simulink model "CoME_ShutOff"  (R2016b)
settings: configuration reference "CodeGenConfigSet" (kept outside this file)
values from neighbouring files (symbols this model uses):
  CoME_drPedHi_C = Calibration.Parameter    [init_CoME_ShutOff.m]    (also in init_CoME_ShutOff_SIL.m = Simulink.Parameter)
  CoME_drPedLo_C = Calibration.Parameter    [init_CoME_ShutOff.m]    (also in init_CoME_ShutOff_SIL.m = Simulink.Parameter)
  CoME_nEng1Hi_C = Calibration.Parameter    [init_CoME_ShutOff.m]    (also in init_CoME_ShutOff_SIL.m = Simulink.Parameter)
  CoME_nEng1Lo_C = Calibration.Parameter    [init_CoME_ShutOff.m]    (also in init_CoME_ShutOff_SIL.m = Simulink.Parameter)
  CoME_nEng2Hi_C = Calibration.Parameter    [init_CoME_ShutOff.m]    (also in init_CoME_ShutOff_SIL.m = Simulink.Parameter)
  CoME_nEng2Lo_C = Calibration.Parameter    [init_CoME_ShutOff.m]    (also in init_CoME_ShutOff_SIL.m = Simulink.Parameter)
  CoME_numTraGearMax_C = Calibration.Parameter    [init_CoME_ShutOff.m]    (also in init_CoME_ShutOff_SIL.m = Simulink.Parameter)
  CoME_pEnv1Hi_C = Calibration.Parameter    [init_CoME_ShutOff.m]    (also in init_CoME_ShutOff_SIL.m = Simulink.Parameter)
  CoME_pEnv1Lo_C = Calibration.Parameter    [init_CoME_ShutOff.m]    (also in init_CoME_ShutOff_SIL.m = Simulink.Parameter)
  CoME_pEnv2Hi_C = Calibration.Parameter    [init_CoME_ShutOff.m]    (also in init_CoME_ShutOff_SIL.m = Simulink.Parameter)
  CoME_pEnv2Lo_C = Calibration.Parameter    [init_CoME_ShutOff.m]    (also in init_CoME_ShutOff_SIL.m = Simulink.Parameter)
  CoME_rPedHi_C = Calibration.Parameter    [init_CoME_ShutOff.m]    (also in init_CoME_ShutOff_SIL.m = Simulink.Parameter)
  CoME_rPedLo_C = Calibration.Parameter    [init_CoME_ShutOff.m]    (also in init_CoME_ShutOff_SIL.m = Simulink.Parameter)
  CoME_stAlt_CW = Calibration.Parameter    [init_CoME_ShutOff.m]    (also in init_CoME_ShutOff_SIL.m = Simulink.Parameter)
  CoME_stEEM_C = Calibration.Parameter    [init_CoME_ShutOff.m]    (also in init_CoME_ShutOff_SIL.m = Simulink.Parameter)
  CoME_stFan_CW = Calibration.Parameter    [init_CoME_ShutOff.m]    (also in init_CoME_ShutOff_SIL.m = Simulink.Parameter)
  CoME_tEnvAir1Hi_C = Calibration.Parameter    [init_CoME_ShutOff.m]    (also in init_CoME_ShutOff_SIL.m = Simulink.Parameter)
  CoME_tEnvAir1Lo_C = Calibration.Parameter    [init_CoME_ShutOff.m]    (also in init_CoME_ShutOff_SIL.m = Simulink.Parameter)
  CoME_tEnvAir2Hi_C = Calibration.Parameter    [init_CoME_ShutOff.m]    (also in init_CoME_ShutOff_SIL.m = Simulink.Parameter)
  CoME_tEnvAir2Lo_C = Calibration.Parameter    [init_CoME_ShutOff.m]    (also in init_CoME_ShutOff_SIL.m = Simulink.Parameter)
  CoME_tiBattVltgOff_C = Calibration.Parameter    [init_CoME_ShutOff.m]    (also in init_CoME_ShutOff_SIL.m = Simulink.Parameter)
  CoME_tiDrvOn_C = Calibration.Parameter    [init_CoME_ShutOff.m]    (also in init_CoME_ShutOff_SIL.m = Simulink.Parameter)
  CoME_tiMaxOffAcc_CUR = Calibration.Parameter    [init_CoME_ShutOff.m]    (also in init_CoME_ShutOff_SIL.m = Simulink.Parameter)
  CoME_tiMaxOffAcc_CURX = Calibration.Parameter    [init_CoME_ShutOff.m]    (also in init_CoME_ShutOff_SIL.m = Simulink.Parameter)
  CoME_tiMaxOffDrvOff_CUR = Calibration.Parameter    [init_CoME_ShutOff.m]    (also in init_CoME_ShutOff_SIL.m = Simulink.Parameter)
  CoME_tiMaxOffDrvOff_CURX = Calibration.Parameter    [init_CoME_ShutOff.m]    (also in init_CoME_ShutOff_SIL.m = Simulink.Parameter)
  CoME_tiMinOffAcc_CUR = Calibration.Parameter    [init_CoME_ShutOff.m]    (also in init_CoME_ShutOff_SIL.m = Simulink.Parameter)
  CoME_tiMinOffAcc_CURX = Calibration.Parameter    [init_CoME_ShutOff.m]    (also in init_CoME_ShutOff_SIL.m = Simulink.Parameter)
  CoME_tiMinOffDrvOff_CUR = Calibration.Parameter    [init_CoME_ShutOff.m]    (also in init_CoME_ShutOff_SIL.m = Simulink.Parameter)
  CoME_tiMinOffDrvOff_CURX = Calibration.Parameter    [init_CoME_ShutOff.m]    (also in init_CoME_ShutOff_SIL.m = Simulink.Parameter)
  CoME_tiOffStrtAC_C = Calibration.Parameter    [init_CoME_ShutOff.m]    (also in init_CoME_ShutOff_SIL.m = Simulink.Parameter)
  CoME_tiOffStrtAlt_C = Calibration.Parameter    [init_CoME_ShutOff.m]    (also in init_CoME_ShutOff_SIL.m = Simulink.Parameter)
  CoME_trqAcc_C = Calibration.Parameter    [init_CoME_ShutOff.m]    (also in init_CoME_ShutOff_SIL.m = Simulink.Parameter)
  CoME_trqACMax_C = Calibration.Parameter    [init_CoME_ShutOff.m]    (also in init_CoME_ShutOff_SIL.m = Simulink.Parameter)
  CoME_trqBattVltg_C = Calibration.Parameter    [init_CoME_ShutOff.m]    (also in init_CoME_ShutOff_SIL.m = Simulink.Parameter)
  CoME_trqDrvOff_C = Calibration.Parameter    [init_CoME_ShutOff.m]    (also in init_CoME_ShutOff_SIL.m = Simulink.Parameter)
  CoME_trqStrt_C = Calibration.Parameter    [init_CoME_ShutOff.m]    (also in init_CoME_ShutOff_SIL.m = Simulink.Parameter)
  CoME_uBattMinHi_C = Calibration.Parameter    [init_CoME_ShutOff.m]    (also in init_CoME_ShutOff_SIL.m = Simulink.Parameter)
  CoME_uBattMinLo_C = Calibration.Parameter    [init_CoME_ShutOff.m]    (also in init_CoME_ShutOff_SIL.m = Simulink.Parameter)
  CoME_vX1Hi_C = Calibration.Parameter    [init_CoME_ShutOff.m]    (also in init_CoME_ShutOff_SIL.m = Simulink.Parameter)
  CoME_vX1Lo_C = Calibration.Parameter    [init_CoME_ShutOff.m]    (also in init_CoME_ShutOff_SIL.m = Simulink.Parameter)
  CoME_vX2Hi_C = Calibration.Parameter    [init_CoME_ShutOff.m]    (also in init_CoME_ShutOff_SIL.m = Simulink.Parameter)
  CoME_vX2Lo_C = Calibration.Parameter    [init_CoME_ShutOff.m]    (also in init_CoME_ShutOff_SIL.m = Simulink.Parameter)
  NUM_WAHT_SY = uint8(0)    [init_CoME_ShutOff.m]    (also in init_CoME_ShutOff_SIL.m)
undefined symbols (not defined in the file or in its folder): CoME_ShutOff_DT, EngState_conv, HPUn_etaPmp_MAPY
libraries: CXLib x32, simulink x8
settings Model: Creator=Colin  LastModifiedBy=wangrui
settings ConfigSetRef: SourceLocation=Base Workspace

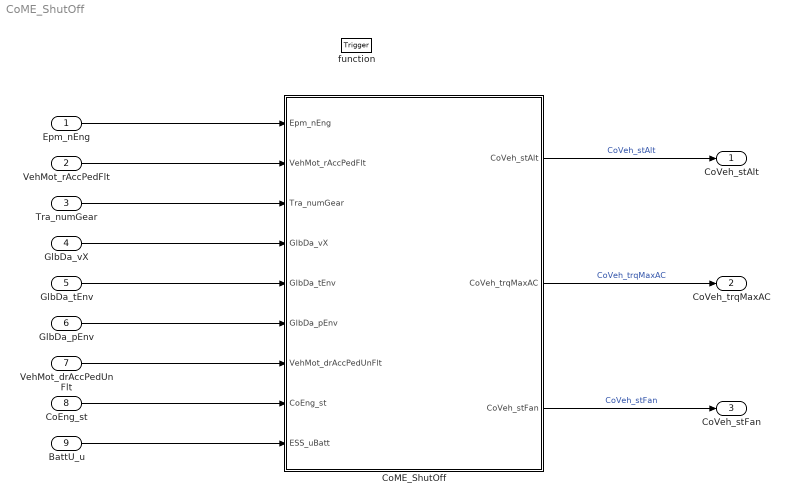
== system CoME_ShutOff ==
  Epm_nEng : Inport  Tag=rpm  Description=Engine speed  OutMin=0  OutMax=6000  OutDataTypeStr=EngSpeed_rpm
  VehMot_rAccPedFlt : Inport  Tag=%  Description=Filtered accelerator pedal value  Port=2  OutMin=0  OutMax=100  OutDataTypeStr=Accpedal_rate
  Tra_numGear : Inport  Description=Current gear information  Port=3  OutMin=-128  OutMax=127  OutDataTypeStr=Tra_num
  GlbDa_vX : Inport  Tag=km/h  Description=Longitudinal vehicle speed (X-direction)  Port=4  OutMin=0  OutMax=250  OutDataTypeStr=VehSpeed_km_h
  GlbDa_tEnv : Inport  Tag=deg  Description=environment temperature  Port=5  OutMin=-50  OutMax=150  OutDataTypeStr=Temp_deg
  GlbDa_pEnv : Inport  Tag=kPa  Description=environmental pressure  Port=6  OutMin=-3000  OutMax=3000  OutDataTypeStr=AirPressure_kPa
  VehMot_drAccPedUnFlt : Inport  Tag=%/s  Description=accelerator pedal angle slope, unfiltered  Port=7  OutMin=-400  OutMax=399  OutDataTypeStr=Accpedal_rate_s
  CoEng_st : Inport  Description=Engine coordinator state  Port=8  OutDataTypeStr=Enum: EngState_conv
  BattU_u : Inport  Tag=mv  Description=Battery voltage  Port=9  OutMin=0  OutMax=50000  OutDataTypeStr=Battery_mv
  function : TriggerPort  TriggerType=function-call  VariantControl=Variant
  CoME_ShutOff : Subsystem  RTWFcnName=CoME_ShutOff_Co  RTWFileName=CoME_ShutOff
      settings: MinAlgLoopOccurrences=on  RTWSystemCode=Nonreusable function  RTWFcnNameOpts=User specified  RTWFileNameOpts=User specified
  CoVeh_stAlt : Outport  Description=Status: Alternator start-up  OutMin=0  OutMax=1  OutDataTypeStr=boolean
  CoVeh_trqMaxAC : Outport  Tag=Nm  Description=Maximum allowed AC torque consumption  Port=2  OutMin=-3000  OutMax=3276.7  OutDataTypeStr=Trq_Nm
  CoVeh_stFan : Outport  Description=Status: Fan start-up  Port=3  OutMin=0  OutMax=1  OutDataTypeStr=boolean
  wires:
  CoME_ShutOff/1(CoVeh_stAlt) -> CoVeh_stAlt/1  "CoVeh_stAlt"
  CoME_ShutOff/2(CoVeh_trqMaxAC) -> CoVeh_trqMaxAC/1  "CoVeh_trqMaxAC"
  CoME_ShutOff/3(CoVeh_stFan) -> CoVeh_stFan/1  "CoVeh_stFan"
  Epm_nEng/1 -> CoME_ShutOff/1(Epm_nEng)
  VehMot_rAccPedFlt/1 -> CoME_ShutOff/2(VehMot_rAccPedFlt)
  Tra_numGear/1 -> CoME_ShutOff/3(Tra_numGear)
  GlbDa_vX/1 -> CoME_ShutOff/4(GlbDa_vX)
  GlbDa_tEnv/1 -> CoME_ShutOff/5(GlbDa_tEnv)
  GlbDa_pEnv/1 -> CoME_ShutOff/6(GlbDa_pEnv)
  VehMot_drAccPedUnFlt/1 -> CoME_ShutOff/7(VehMot_drAccPedUnFlt)
  CoEng_st/1 -> CoME_ShutOff/8(CoEng_st)
  BattU_u/1 -> CoME_ShutOff/9(ESS_uBatt)

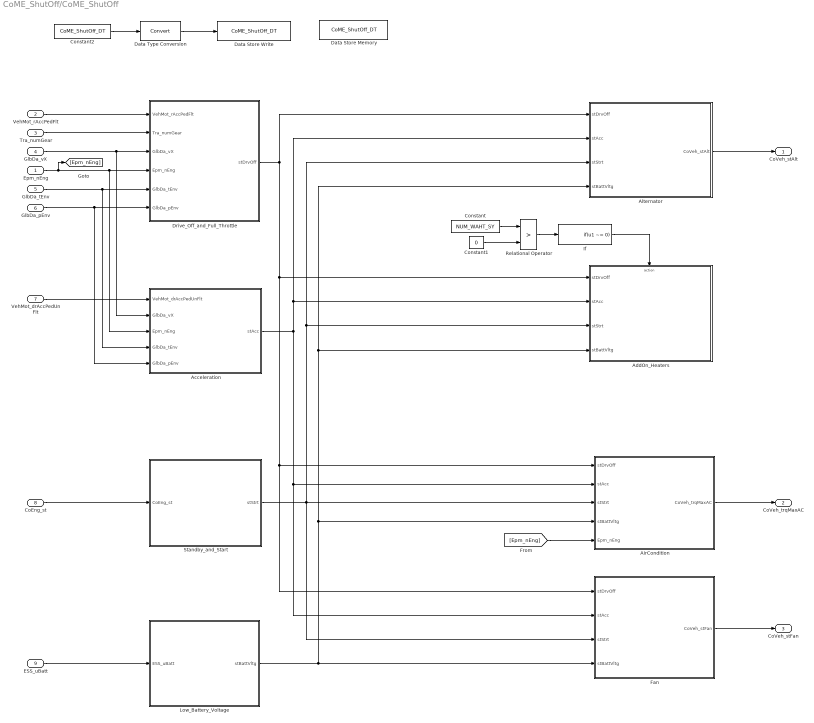
== system CoME_ShutOff/CoME_ShutOff ==
  Epm_nEng : Inport
  VehMot_rAccPedFlt : Inport  Port=2
  Tra_numGear : Inport  Port=3
  GlbDa_vX : Inport  Port=4
  GlbDa_tEnv : Inport  Port=5
  GlbDa_pEnv : Inport  Port=6
  VehMot_drAccPedUnFlt : Inport  Port=7
  CoEng_st : Inport  Port=8
  ESS_uBatt : Inport  Port=9
  Acceleration : Subsystem
  AddOn_Heaters : Subsystem  TreatAsAtomicUnit=on
  AirCondition : Subsystem
      settings: MinAlgLoopOccurrences=on
  Alternator : Subsystem
  Constant : Constant  Value=NUM_WAHT_SY  OutDataTypeStr=uint8
  Constant1 : Constant  Value=0  OutDataTypeStr=Inherit: Inherit via back propagation
  Constant2 : Constant  Value=CoME_ShutOff_DT
  Data Store Memory : DataStoreMemory  DataStoreName=CoME_ShutOff_DT  ReadBeforeWriteMsg=warning  WriteAfterWriteMsg=warning  WriteAfterReadMsg=warning  InitialValue=10  ShowAdditionalParam=off  OutDataTypeStr=EngTime_ms
  Data Store Write : DataStoreWrite  DataStoreName=CoME_ShutOff_DT
  Data Type Conversion : DataTypeConversion
  Drive_Off_and_Full_Throttle : Subsystem
  Fan : Subsystem
  If : If  IfExpression=u1 ~= 0  ShowElse=off
  Low_Battery_Voltage : Subsystem
  Relational Operator : RelationalOperator  Operator=>  OutDataTypeStr=boolean  RndMeth=Simplest  InputSameDT=on
  Standby_and_Start : Subsystem
  CoVeh_stAlt : Outport
  CoVeh_trqMaxAC : Outport  Port=2
  CoVeh_stFan : Outport  Port=3
  wires:
  Epm_nEng/1 -> [Epm_nEng], Drive_Off_and_Full_Throttle/4(Epm_nEng), Acceleration/3(Epm_nEng)
  VehMot_rAccPedFlt/1 -> Drive_Off_and_Full_Throttle/1(VehMot_rAccPedFlt)
  ESS_uBatt/1 -> Low_Battery_Voltage/1(ESS_uBatt)
  GlbDa_pEnv/1 -> Drive_Off_and_Full_Throttle/6(GlbDa_pEnv), Acceleration/5(GlbDa_pEnv)
  GlbDa_tEnv/1 -> Drive_Off_and_Full_Throttle/5(GlbDa_tEnv), Acceleration/4(GlbDa_tEnv)
  GlbDa_vX/1 -> Drive_Off_and_Full_Throttle/3(GlbDa_vX), Acceleration/2(GlbDa_vX)
  Tra_numGear/1 -> Drive_Off_and_Full_Throttle/2(Tra_numGear)
  VehMot_drAccPedUnFlt/1 -> Acceleration/1(VehMot_drAccPedUnFlt)
  AirCondition/1(CoVeh_trqMaxAC) -> CoVeh_trqMaxAC/1
  Fan/1(CoVeh_stFan) -> CoVeh_stFan/1
  CoEng_st/1 -> Standby_and_Start/1(CoEng_st)
  [Epm_nEng] -> AirCondition/5(Epm_nEng)
  Low_Battery_Voltage/1(stBattVltg) -> Fan/4(stBattVltg), AirCondition/4(stBattVltg), AddOn_Heaters/4(stBattVltg), Alternator/4(stBattVltg)
  Drive_Off_and_Full_Throttle/1(stDrvOff) -> Alternator/1(stDrvOff), AirCondition/1(stDrvOff), Fan/1(stDrvOff), AddOn_Heaters/1(stDrvOff)
  Standby_and_Start/1(stStrt) -> AirCondition/3(stStrt), AddOn_Heaters/3(stStrt), Alternator/3(stStrt), Fan/3(stStrt)
  Acceleration/1(stAcc) -> Alternator/2(stAcc), AddOn_Heaters/2(stAcc), AirCondition/2(stAcc), Fan/2(stAcc)
  Alternator/1(CoVeh_stAlt) -> CoVeh_stAlt/1
  Constant1/1 -> Relational Operator/2
  If/1 -> AddOn_Heaters/Action
  Constant/1 -> Relational Operator/1
  Relational Operator/1 -> If/1
  Constant2/1 -> Data Type Conversion/1
  Data Type Conversion/1 -> Data Store Write/1

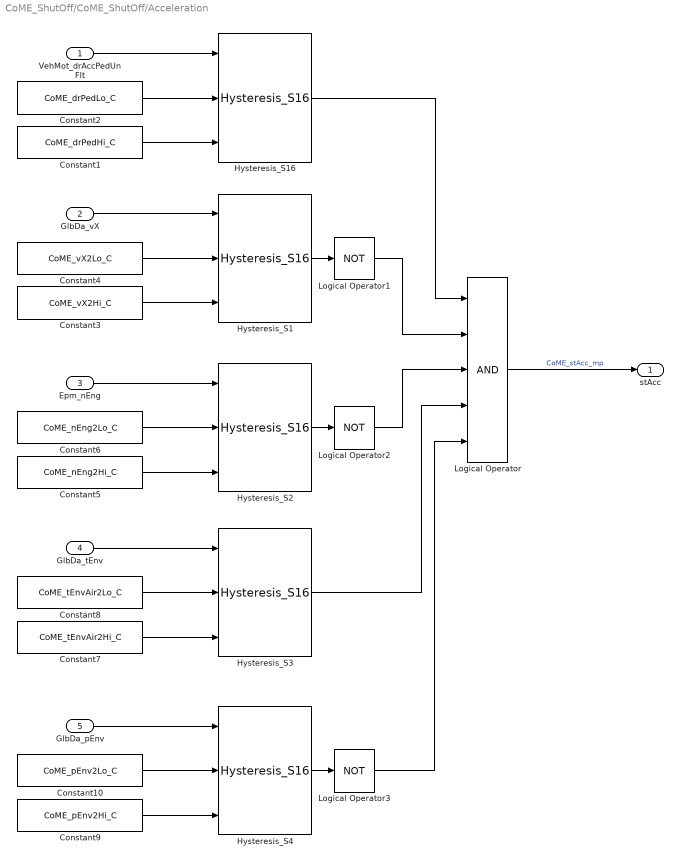
== system CoME_ShutOff/CoME_ShutOff/Acceleration ==
  VehMot_drAccPedUnFlt : Inport
  GlbDa_vX : Inport  Port=2
  Epm_nEng : Inport  Port=3
  GlbDa_tEnv : Inport  Port=4
  GlbDa_pEnv : Inport  Port=5
  Constant1 : Constant  Value=CoME_drPedHi_C
  Constant10 : Constant  Value=CoME_pEnv2Lo_C
  Constant2 : Constant  Value=CoME_drPedLo_C
  Constant3 : Constant  Value=CoME_vX2Hi_C
  Constant4 : Constant  Value=CoME_vX2Lo_C
  Constant5 : Constant  Value=CoME_nEng2Hi_C
  Constant6 : Constant  Value=CoME_nEng2Lo_C
  Constant7 : Constant  Value=CoME_tEnvAir2Hi_C
  Constant8 : Constant  Value=CoME_tEnvAir2Lo_C
  Constant9 : Constant  Value=CoME_pEnv2Hi_C
  Hysteresis_S{1..4,16} (5 alike) : CXLib/Hysteresis_S16
  Logical Operator : Logic  Inputs=5  OutDataTypeStr=boolean
  Logical Operator1 : Logic  Operator=NOT  OutDataTypeStr=boolean
  Logical Operator2 : Logic  Operator=NOT  OutDataTypeStr=boolean
  Logical Operator3 : Logic  Operator=NOT  OutDataTypeStr=boolean
  stAcc : Outport
  wires:
  Hysteresis_S16/1 -> Logical Operator/1
  Logical Operator1/1 -> Logical Operator/2
  Logical Operator2/1 -> Logical Operator/3
  Hysteresis_S3/1 -> Logical Operator/4
  Logical Operator3/1 -> Logical Operator/5
  Hysteresis_S4/1 -> Logical Operator3/1
  Hysteresis_S2/1 -> Logical Operator2/1
  Hysteresis_S1/1 -> Logical Operator1/1
  GlbDa_pEnv/1 -> Hysteresis_S4/1
  Constant10/1 -> Hysteresis_S4/2
  Constant9/1 -> Hysteresis_S4/3
  GlbDa_tEnv/1 -> Hysteresis_S3/1
  Constant8/1 -> Hysteresis_S3/2
  Constant7/1 -> Hysteresis_S3/3
  Epm_nEng/1 -> Hysteresis_S2/1
  Constant6/1 -> Hysteresis_S2/2
  Constant5/1 -> Hysteresis_S2/3
  GlbDa_vX/1 -> Hysteresis_S1/1
  Constant4/1 -> Hysteresis_S1/2
  Constant3/1 -> Hysteresis_S1/3
  Constant1/1 -> Hysteresis_S16/3
  Constant2/1 -> Hysteresis_S16/2
  VehMot_drAccPedUnFlt/1 -> Hysteresis_S16/1
  Logical Operator/1 -> stAcc/1  "CoME_stAcc_mp"

== system CoME_ShutOff/CoME_ShutOff/AddOn_Heaters ==
  note: %文档中没有图或文字描述%
  stDrvOff : Inport
  stAcc : Inport  Port=2
  stStrt : Inport  Port=3
  stBattVltg : Inport  Port=4
  Action Port : ActionPort  ActionType=then
  Terminator{,1..3} (4 alike) : Terminator
  wires:
  stBattVltg/1 -> Terminator3/1
  stStrt/1 -> Terminator2/1
  stAcc/1 -> Terminator1/1
  stDrvOff/1 -> Terminator/1

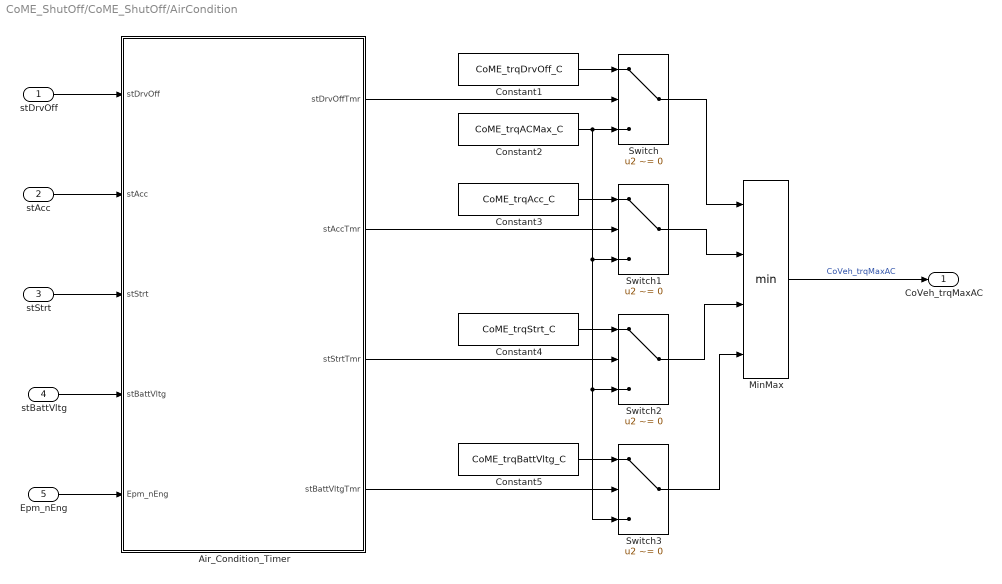
== system CoME_ShutOff/CoME_ShutOff/AirCondition ==
  stDrvOff : Inport
  stAcc : Inport  Port=2
  stStrt : Inport  Port=3
  stBattVltg : Inport  Port=4
  Epm_nEng : Inport  Port=5
  Air_Condition_Timer : Subsystem
  Constant1 : Constant  Value=CoME_trqDrvOff_C
  Constant2 : Constant  Value=CoME_trqACMax_C
  Constant3 : Constant  Value=CoME_trqAcc_C
  Constant4 : Constant  Value=CoME_trqStrt_C
  Constant5 : Constant  Value=CoME_trqBattVltg_C
  MinMax : MinMax  Inputs=4  InputSameDT=on
  Switch{,1..3} (4 alike) : Switch  Criteria=u2 ~= 0  InputSameDT=on
  CoVeh_trqMaxAC : Outport
  wires:
  Epm_nEng/1 -> Air_Condition_Timer/5(Epm_nEng)
  stDrvOff/1 -> Air_Condition_Timer/1(stDrvOff)
  stAcc/1 -> Air_Condition_Timer/2(stAcc)
  stStrt/1 -> Air_Condition_Timer/3(stStrt)
  stBattVltg/1 -> Air_Condition_Timer/4(stBattVltg)
  Air_Condition_Timer/4(stBattVltgTmr) -> Switch3/2
  Air_Condition_Timer/3(stStrtTmr) -> Switch2/2
  Air_Condition_Timer/2(stAccTmr) -> Switch1/2
  Air_Condition_Timer/1(stDrvOffTmr) -> Switch/2
  Constant5/1 -> Switch3/1
  Constant4/1 -> Switch2/1
  Constant3/1 -> Switch1/1
  Constant1/1 -> Switch/1
  Constant2/1 -> Switch/3, Switch1/3, Switch3/3, Switch2/3
  Switch/1 -> MinMax/1
  Switch1/1 -> MinMax/2
  Switch2/1 -> MinMax/3
  Switch3/1 -> MinMax/4
  MinMax/1 -> CoVeh_trqMaxAC/1  "CoVeh_trqMaxAC"

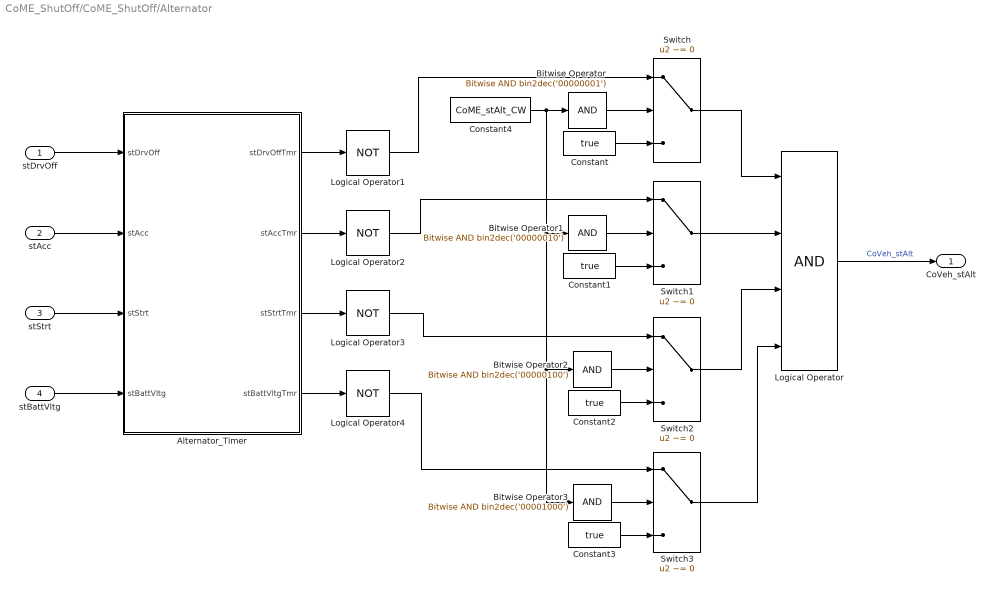
== system CoME_ShutOff/CoME_ShutOff/Alternator ==
  stDrvOff : Inport
  stAcc : Inport  Port=2
  stStrt : Inport  Port=3
  stBattVltg : Inport  Port=4
  Alternator_Timer : Subsystem
  Bitwise Operator : simulink/Logic and Bit Operations/Bitwise Operator  logicop=AND  UseBitMask=on  BitMask=bin2dec('00000001')  BitMaskRealWorld=Stored Integer
  Bitwise Operator1 : simulink/Logic and Bit Operations/Bitwise Operator  logicop=AND  UseBitMask=on  BitMask=bin2dec('00000010')  BitMaskRealWorld=Stored Integer
  Bitwise Operator2 : simulink/Logic and Bit Operations/Bitwise Operator  logicop=AND  UseBitMask=on  BitMask=bin2dec('00000100')  BitMaskRealWorld=Stored Integer
  Bitwise Operator3 : simulink/Logic and Bit Operations/Bitwise Operator  logicop=AND  UseBitMask=on  BitMask=bin2dec('00001000')  BitMaskRealWorld=Stored Integer
  Constant{,1..3} (4 alike) : Constant  Value=true  OutDataTypeStr=boolean
  Constant4 : Constant  Value=CoME_stAlt_CW
  Logical Operator : Logic  Inputs=4  OutDataTypeStr=boolean
  Logical Operator{1..4} (4 alike) : Logic  Operator=NOT  OutDataTypeStr=boolean
  Switch{,1..3} (4 alike) : Switch  Criteria=u2 ~= 0  InputSameDT=on
  CoVeh_stAlt : Outport
  wires:
  Logical Operator4/1 -> Switch3/1
  Bitwise Operator3/1 -> Switch3/2
  Logical Operator3/1 -> Switch2/1
  Bitwise Operator2/1 -> Switch2/2
  Logical Operator2/1 -> Switch1/1
  Bitwise Operator1/1 -> Switch1/2
  Logical Operator1/1 -> Switch/1
  Constant4/1 -> Bitwise Operator1/1, Bitwise Operator2/1, Bitwise Operator3/1, Bitwise Operator/1
  Bitwise Operator/1 -> Switch/2
  Constant3/1 -> Switch3/3
  Constant2/1 -> Switch2/3
  Constant1/1 -> Switch1/3
  Constant/1 -> Switch/3
  Switch3/1 -> Logical Operator/4
  Switch2/1 -> Logical Operator/3
  Switch1/1 -> Logical Operator/2
  Switch/1 -> Logical Operator/1
  Logical Operator/1 -> CoVeh_stAlt/1  "CoVeh_stAlt"
  Alternator_Timer/4(stBattVltgTmr) -> Logical Operator4/1
  Alternator_Timer/3(stStrtTmr) -> Logical Operator3/1
  Alternator_Timer/2(stAccTmr) -> Logical Operator2/1
  Alternator_Timer/1(stDrvOffTmr) -> Logical Operator1/1
  stBattVltg/1 -> Alternator_Timer/4(stBattVltg)
  stStrt/1 -> Alternator_Timer/3(stStrt)
  stAcc/1 -> Alternator_Timer/2(stAcc)
  stDrvOff/1 -> Alternator_Timer/1(stDrvOff)

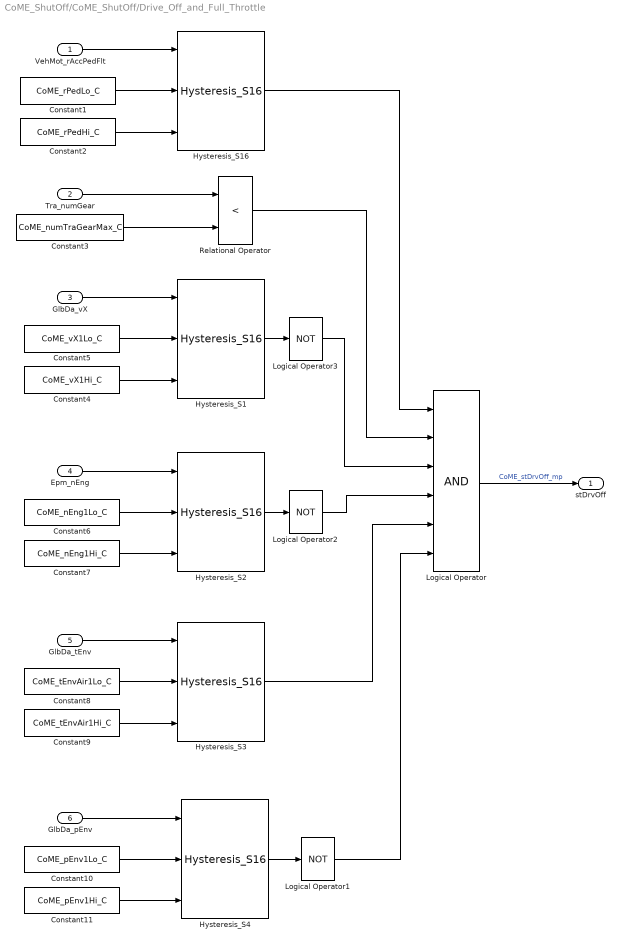
== system CoME_ShutOff/CoME_ShutOff/Drive_Off_and_Full_Throttle ==
  VehMot_rAccPedFlt : Inport
  Tra_numGear : Inport  Port=2
  GlbDa_vX : Inport  Port=3
  Epm_nEng : Inport  Port=4
  GlbDa_tEnv : Inport  Port=5
  GlbDa_pEnv : Inport  Port=6
  Constant1 : Constant  Value=CoME_rPedLo_C
  Constant10 : Constant  Value=CoME_pEnv1Lo_C
  Constant11 : Constant  Value=CoME_pEnv1Hi_C
  Constant2 : Constant  Value=CoME_rPedHi_C
  Constant3 : Constant  Value=CoME_numTraGearMax_C
  Constant4 : Constant  Value=CoME_vX1Hi_C
  Constant5 : Constant  Value=CoME_vX1Lo_C
  Constant6 : Constant  Value=CoME_nEng1Lo_C
  Constant7 : Constant  Value=CoME_nEng1Hi_C
  Constant8 : Constant  Value=CoME_tEnvAir1Lo_C
  Constant9 : Constant  Value=CoME_tEnvAir1Hi_C
  Hysteresis_S{1..4,16} (5 alike) : CXLib/Hysteresis_S16
  Logical Operator : Logic  Inputs=6  OutDataTypeStr=boolean
  Logical Operator1 : Logic  Operator=NOT  OutDataTypeStr=boolean
  Logical Operator2 : Logic  Operator=NOT  OutDataTypeStr=boolean
  Logical Operator3 : Logic  Operator=NOT  OutDataTypeStr=boolean
  Relational Operator : RelationalOperator  Operator=<  OutDataTypeStr=boolean  RndMeth=Simplest  InputSameDT=on
  stDrvOff : Outport
  wires:
  Constant10/1 -> Hysteresis_S4/2
  Constant11/1 -> Hysteresis_S4/3
  GlbDa_pEnv/1 -> Hysteresis_S4/1
  Constant9/1 -> Hysteresis_S3/3
  Constant8/1 -> Hysteresis_S3/2
  GlbDa_tEnv/1 -> Hysteresis_S3/1
  Constant7/1 -> Hysteresis_S2/3
  Constant6/1 -> Hysteresis_S2/2
  Epm_nEng/1 -> Hysteresis_S2/1
  GlbDa_vX/1 -> Hysteresis_S1/1
  Constant5/1 -> Hysteresis_S1/2
  Constant4/1 -> Hysteresis_S1/3
  Logical Operator3/1 -> Logical Operator/3
  Hysteresis_S1/1 -> Logical Operator3/1
  Logical Operator2/1 -> Logical Operator/4
  Hysteresis_S2/1 -> Logical Operator2/1
  Hysteresis_S3/1 -> Logical Operator/5
  Logical Operator1/1 -> Logical Operator/6
  Hysteresis_S4/1 -> Logical Operator1/1
  Tra_numGear/1 -> Relational Operator/1
  Constant3/1 -> Relational Operator/2
  Relational Operator/1 -> Logical Operator/2
  Constant2/1 -> Hysteresis_S16/3
  Constant1/1 -> Hysteresis_S16/2
  VehMot_rAccPedFlt/1 -> Hysteresis_S16/1
  Hysteresis_S16/1 -> Logical Operator/1
  Logical Operator/1 -> stDrvOff/1  "CoME_stDrvOff_mp"

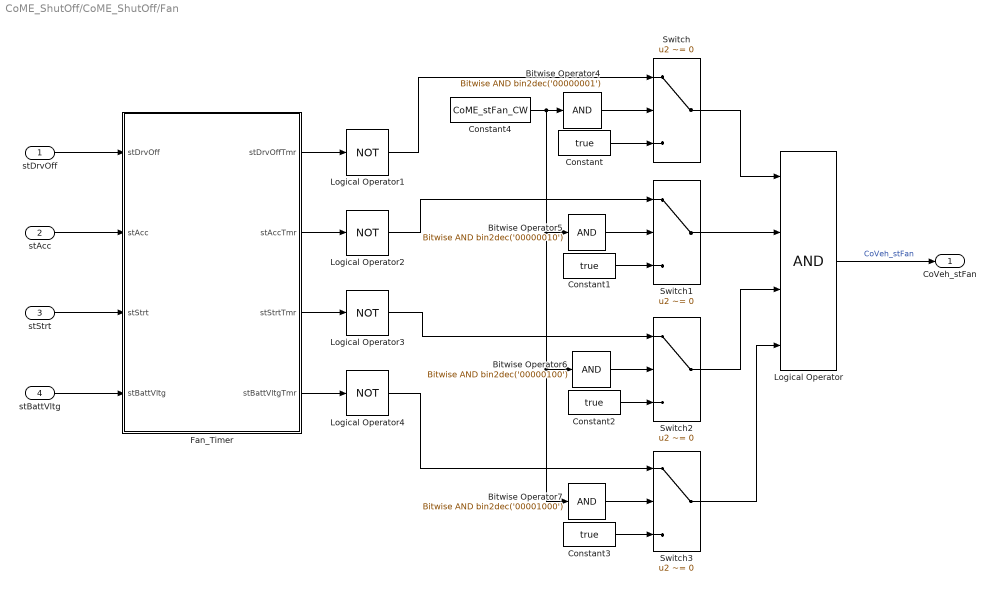
== system CoME_ShutOff/CoME_ShutOff/Fan ==
  stDrvOff : Inport
  stAcc : Inport  Port=2
  stStrt : Inport  Port=3
  stBattVltg : Inport  Port=4
  Bitwise Operator4 : simulink/Logic and Bit Operations/Bitwise Operator  logicop=AND  UseBitMask=on  BitMask=bin2dec('00000001')  BitMaskRealWorld=Stored Integer
  Bitwise Operator5 : simulink/Logic and Bit Operations/Bitwise Operator  logicop=AND  UseBitMask=on  BitMask=bin2dec('00000010')  BitMaskRealWorld=Stored Integer
  Bitwise Operator6 : simulink/Logic and Bit Operations/Bitwise Operator  logicop=AND  UseBitMask=on  BitMask=bin2dec('00000100')  BitMaskRealWorld=Stored Integer
  Bitwise Operator7 : simulink/Logic and Bit Operations/Bitwise Operator  logicop=AND  UseBitMask=on  BitMask=bin2dec('00001000')  BitMaskRealWorld=Stored Integer
  Constant{,1..3} (4 alike) : Constant  Value=true  OutDataTypeStr=boolean
  Constant4 : Constant  Value=CoME_stFan_CW
  Fan_Timer : Subsystem
  Logical Operator : Logic  Inputs=4  OutDataTypeStr=boolean
  Logical Operator{1..4} (4 alike) : Logic  Operator=NOT  OutDataTypeStr=boolean
  Switch{,1..3} (4 alike) : Switch  Criteria=u2 ~= 0  InputSameDT=on
  CoVeh_stFan : Outport
  wires:
  Logical Operator4/1 -> Switch3/1
  Bitwise Operator7/1 -> Switch3/2
  Logical Operator3/1 -> Switch2/1
  Bitwise Operator6/1 -> Switch2/2
  Logical Operator2/1 -> Switch1/1
  Bitwise Operator5/1 -> Switch1/2
  Logical Operator1/1 -> Switch/1
  Constant4/1 -> Bitwise Operator5/1, Bitwise Operator6/1, Bitwise Operator7/1, Bitwise Operator4/1
  Bitwise Operator4/1 -> Switch/2
  Constant3/1 -> Switch3/3
  Constant2/1 -> Switch2/3
  Constant1/1 -> Switch1/3
  Constant/1 -> Switch/3
  Switch3/1 -> Logical Operator/4
  Switch2/1 -> Logical Operator/3
  Switch1/1 -> Logical Operator/2
  Switch/1 -> Logical Operator/1
  Logical Operator/1 -> CoVeh_stFan/1  "CoVeh_stFan"
  Fan_Timer/4(stBattVltgTmr) -> Logical Operator4/1
  Fan_Timer/3(stStrtTmr) -> Logical Operator3/1
  Fan_Timer/2(stAccTmr) -> Logical Operator2/1
  Fan_Timer/1(stDrvOffTmr) -> Logical Operator1/1
  stBattVltg/1 -> Fan_Timer/4(stBattVltg)
  stStrt/1 -> Fan_Timer/3(stStrt)
  stAcc/1 -> Fan_Timer/2(stAcc)
  stDrvOff/1 -> Fan_Timer/1(stDrvOff)

== system CoME_ShutOff/CoME_ShutOff/Low_Battery_Voltage ==
  ESS_uBatt : Inport
  Constant1 : Constant  Value=CoME_uBattMinHi_C
  Constant2 : Constant  Value=CoME_uBattMinLo_C
  Electrical_Energy : Subsystem
  Hysteresis_S16 : CXLib/Hysteresis_S16
  Logical Operator1 : Logic  Operator=NOT  AllPortsSameDT=off  OutDataTypeStr=boolean
  stBattVltg : Outport
  wires:
  Constant1/1 -> Hysteresis_S16/3
  Constant2/1 -> Hysteresis_S16/2
  ESS_uBatt/1 -> Hysteresis_S16/1
  Electrical_Energy/1(stBattVltg) -> stBattVltg/1  "CoME_stBattVltg_mp"
  Logical Operator1/1 -> Electrical_Energy/1(stUBatt)
  Hysteresis_S16/1 -> Logical Operator1/1

== system CoME_ShutOff/CoME_ShutOff/Standby_and_Start ==
  CoEng_st : Inport
  Constant1 : Constant  Value=EngState_conv.COENG_READY
  Constant2 : Constant  Value=EngState_conv.COENG_CRANKING
  Constant3 : Constant  Value=EngState_conv.COENG_STANDBY
  Logical Operator : Logic  Operator=OR  Inputs=3  OutDataTypeStr=boolean
  Relational Operator : RelationalOperator  Operator===  OutDataTypeStr=boolean  RndMeth=Simplest  InputSameDT=on
  Relational Operator1 : RelationalOperator  Operator===  OutDataTypeStr=boolean  RndMeth=Simplest  InputSameDT=on
  Relational Operator2 : RelationalOperator  Operator===  OutDataTypeStr=boolean  RndMeth=Simplest  InputSameDT=on
  stStrt : Outport
  wires:
  Constant3/1 -> Relational Operator2/2
  Constant1/1 -> Relational Operator1/2
  Constant2/1 -> Relational Operator/2
  CoEng_st/1 -> Relational Operator/1, Relational Operator1/1, Relational Operator2/1
  Relational Operator/1 -> Logical Operator/1
  Relational Operator2/1 -> Logical Operator/3
  Relational Operator1/1 -> Logical Operator/2
  Logical Operator/1 -> stStrt/1  "CoME_stStrt_mp"

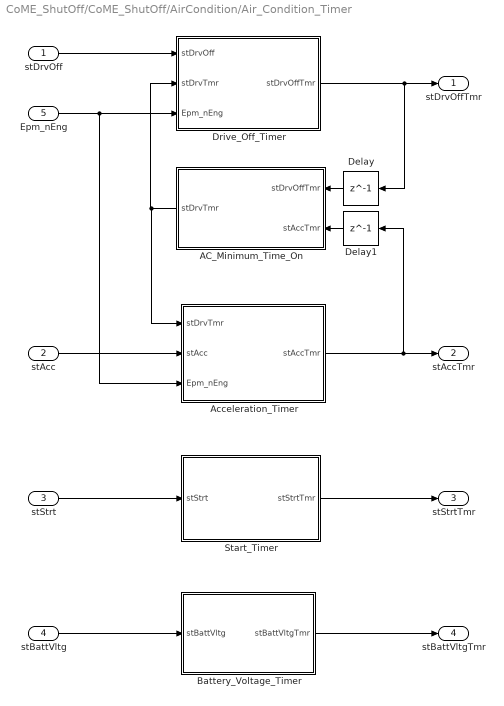
== system CoME_ShutOff/CoME_ShutOff/AirCondition/Air_Condition_Timer ==
  stDrvOff : Inport
  stAcc : Inport  Port=2
  stStrt : Inport  Port=3
  stBattVltg : Inport  Port=4
  Epm_nEng : Inport  Port=5
  AC_Minimum_Time_On : Subsystem
  Acceleration_Timer : Subsystem
  Battery_Voltage_Timer : Subsystem
  Delay : Delay  DelayLength=1  InitialCondition=0
  Delay1 : Delay  DelayLength=1  InitialCondition=0
  Drive_Off_Timer : Subsystem
  Start_Timer : Subsystem
  stDrvOffTmr : Outport
  stAccTmr : Outport  Port=2
  stStrtTmr : Outport  Port=3
  stBattVltgTmr : Outport  Port=4
  wires:
  Delay1/1 -> AC_Minimum_Time_On/2(stAccTmr)
  Delay/1 -> AC_Minimum_Time_On/1(stDrvOffTmr)
  Epm_nEng/1 -> Drive_Off_Timer/3(Epm_nEng), Acceleration_Timer/3(Epm_nEng)
  Battery_Voltage_Timer/1(stBattVltgTmr) -> stBattVltgTmr/1
  stBattVltg/1 -> Battery_Voltage_Timer/1(stBattVltg)
  stStrt/1 -> Start_Timer/1(stStrt)
  Start_Timer/1(stStrtTmr) -> stStrtTmr/1
  stAcc/1 -> Acceleration_Timer/2(stAcc)
  Acceleration_Timer/1(stAccTmr) -> Delay1/1, stAccTmr/1
  AC_Minimum_Time_On/1(stDrvTmr) -> Drive_Off_Timer/2(stDrvTmr), Acceleration_Timer/1(stDrvTmr)
  Drive_Off_Timer/1(stDrvOffTmr) -> stDrvOffTmr/1, Delay/1
  stDrvOff/1 -> Drive_Off_Timer/1(stDrvOff)

== system CoME_ShutOff/CoME_ShutOff/Alternator/Alternator_Timer ==
  stDrvOff : Inport
  stAcc : Inport  Port=2
  stStrt : Inport  Port=3
  stBattVltg : Inport  Port=4
  Constant1 : Constant  Value=1000  OutDataTypeStr=int16
  Constant2 : Constant  Value=CoME_tiOffStrtAlt_C
  Data Store Read : DataStoreRead  DataStoreName=CoME_ShutOff_DT
  Divide : Product  Inputs=**  OutDataTypeStr=EngTime_ms  SaturateOnIntegerOverflow=on
  TurnOffDelay : CXLib/TurnOffDelay
  stDrvOffTmr : Outport
  stAccTmr : Outport  Port=2
  stStrtTmr : Outport  Port=3
  stBattVltgTmr : Outport  Port=4
  wires:
  Constant1/1 -> Divide/2
  Constant2/1 -> Divide/1
  Data Store Read/1 -> TurnOffDelay/3
  stStrt/1 -> TurnOffDelay/1
  TurnOffDelay/1 -> stStrtTmr/1
  stAcc/1 -> stAccTmr/1
  stDrvOff/1 -> stDrvOffTmr/1
  stBattVltg/1 -> stBattVltgTmr/1
  Divide/1 -> TurnOffDelay/2

== system CoME_ShutOff/CoME_ShutOff/Fan/Fan_Timer ==
  stDrvOff : Inport
  stAcc : Inport  Port=2
  stStrt : Inport  Port=3
  stBattVltg : Inport  Port=4
  stDrvOffTmr : Outport
  stAccTmr : Outport  Port=2
  stStrtTmr : Outport  Port=3
  stBattVltgTmr : Outport  Port=4
  wires:
  stStrt/1 -> stStrtTmr/1
  stAcc/1 -> stAccTmr/1
  stDrvOff/1 -> stDrvOffTmr/1
  stBattVltg/1 -> stBattVltgTmr/1

== system CoME_ShutOff/CoME_ShutOff/Low_Battery_Voltage/Electrical_Energy ==
  stUBatt : Inport
  Constant2 : Constant  Value=CoME_stEEM_C
  Logical Operator : Logic  Operator=OR  OutDataTypeStr=boolean
  stBattVltg : Outport
  wires:
  Constant2/1 -> Logical Operator/2
  stUBatt/1 -> Logical Operator/1
  Logical Operator/1 -> stBattVltg/1

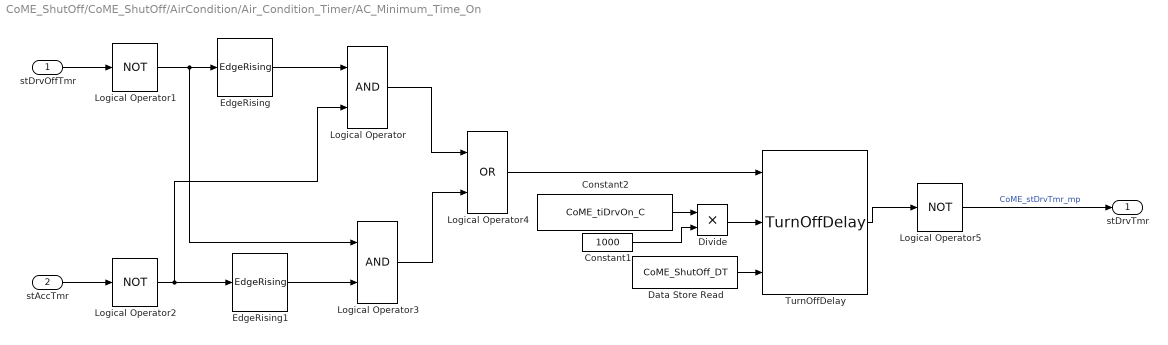
== system CoME_ShutOff/CoME_ShutOff/AirCondition/Air_Condition_Timer/AC_Minimum_Time_On ==
  stDrvOffTmr : Inport
  stAccTmr : Inport  Port=2
  Constant1 : Constant  Value=1000  OutDataTypeStr=int16
  Constant2 : Constant  Value=CoME_tiDrvOn_C
  Data Store Read : DataStoreRead  DataStoreName=CoME_ShutOff_DT
  Divide : Product  Inputs=**  OutDataTypeStr=EngTime_ms  SaturateOnIntegerOverflow=on
  EdgeRising : CXLib/EdgeRising
  EdgeRising1 : CXLib/EdgeRising
  Logical Operator : Logic  OutDataTypeStr=boolean
  Logical Operator1 : Logic  Operator=NOT  OutDataTypeStr=boolean
  Logical Operator2 : Logic  Operator=NOT  OutDataTypeStr=boolean
  Logical Operator3 : Logic  OutDataTypeStr=boolean
  Logical Operator4 : Logic  Operator=OR  OutDataTypeStr=boolean
  Logical Operator5 : Logic  Operator=NOT  OutDataTypeStr=boolean
  TurnOffDelay : CXLib/TurnOffDelay
  stDrvTmr : Outport
  wires:
  Constant1/1 -> Divide/2
  Constant2/1 -> Divide/1
  Divide/1 -> TurnOffDelay/2
  Data Store Read/1 -> TurnOffDelay/3
  Logical Operator5/1 -> stDrvTmr/1  "CoME_stDrvTmr_mp"
  TurnOffDelay/1 -> Logical Operator5/1
  Logical Operator4/1 -> TurnOffDelay/1
  Logical Operator3/1 -> Logical Operator4/2
  Logical Operator/1 -> Logical Operator4/1
  EdgeRising1/1 -> Logical Operator3/2
  Logical Operator2/1 -> Logical Operator/2, EdgeRising1/1
  stAccTmr/1 -> Logical Operator2/1
  EdgeRising/1 -> Logical Operator/1
  Logical Operator1/1 -> EdgeRising/1, Logical Operator3/1
  stDrvOffTmr/1 -> Logical Operator1/1

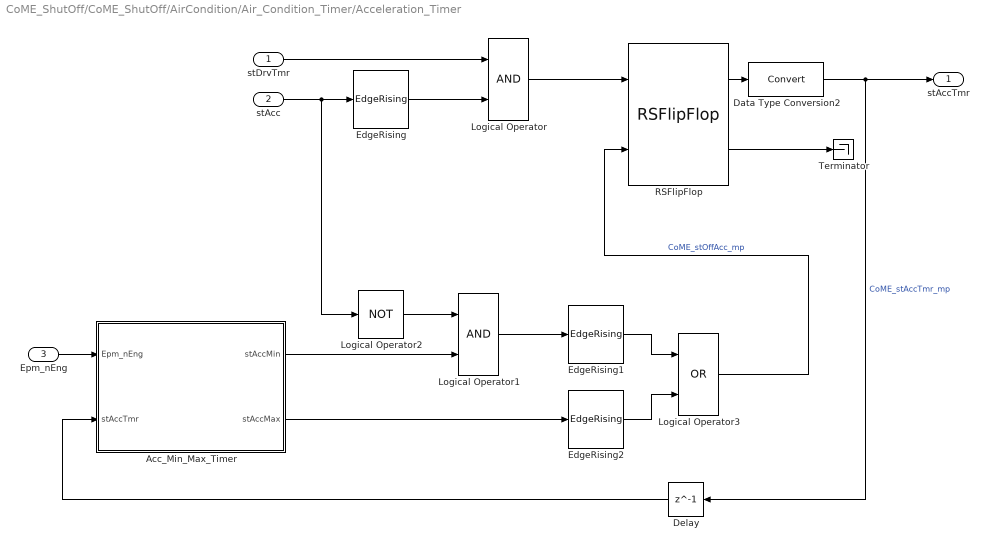
== system CoME_ShutOff/CoME_ShutOff/AirCondition/Air_Condition_Timer/Acceleration_Timer ==
  stDrvTmr : Inport
  stAcc : Inport  Port=2
  Epm_nEng : Inport  Port=3
  Acc_Min_Max_Timer : Subsystem
  Data Type Conversion2 : DataTypeConversion
  Delay : Delay  DelayLength=1  InitialCondition=0
  EdgeRising : CXLib/EdgeRising
  EdgeRising1 : CXLib/EdgeRising
  EdgeRising2 : CXLib/EdgeRising
  Logical Operator : Logic  OutDataTypeStr=boolean
  Logical Operator1 : Logic  OutDataTypeStr=boolean
  Logical Operator2 : Logic  Operator=NOT  OutDataTypeStr=boolean
  Logical Operator3 : Logic  Operator=OR  OutDataTypeStr=boolean
  RSFlipFlop : CXLib/RSFlipFlop
  Terminator : Terminator
  stAccTmr : Outport
  wires:
  Delay/1 -> Acc_Min_Max_Timer/2(stAccTmr)
  Data Type Conversion2/1 -> Delay/1, stAccTmr/1  "CoME_stAccTmr_mp"
  Epm_nEng/1 -> Acc_Min_Max_Timer/1(Epm_nEng)
  Logical Operator3/1 -> RSFlipFlop/2  "CoME_stOffAcc_mp"
  EdgeRising2/1 -> Logical Operator3/2
  EdgeRising1/1 -> Logical Operator3/1
  Acc_Min_Max_Timer/2(stAccMax) -> EdgeRising2/1
  Logical Operator1/1 -> EdgeRising1/1
  Logical Operator2/1 -> Logical Operator1/1
  Acc_Min_Max_Timer/1(stAccMin) -> Logical Operator1/2
  RSFlipFlop/2 -> Terminator/1
  RSFlipFlop/1 -> Data Type Conversion2/1
  Logical Operator/1 -> RSFlipFlop/1
  stDrvTmr/1 -> Logical Operator/1
  EdgeRising/1 -> Logical Operator/2
  stAcc/1 -> EdgeRising/1, Logical Operator2/1

== system CoME_ShutOff/CoME_ShutOff/AirCondition/Air_Condition_Timer/Battery_Voltage_Timer ==
  stBattVltg : Inport
  Constant1 : Constant  Value=1000  OutDataTypeStr=int16
  Constant2 : Constant  Value=CoME_tiBattVltgOff_C
  Data Store Read : DataStoreRead  DataStoreName=CoME_ShutOff_DT
  Divide : Product  Inputs=**  OutDataTypeStr=Inherit: Inherit via back propagation  SaturateOnIntegerOverflow=on
  EdgeRising : CXLib/EdgeRising
  Logical Operator : Logic  Operator=OR  OutDataTypeStr=boolean
  TurnOffDelay : CXLib/TurnOffDelay
  stBattVltgTmr : Outport
  wires:
  Constant1/1 -> Divide/2
  Constant2/1 -> Divide/1
  Divide/1 -> TurnOffDelay/2
  Data Store Read/1 -> TurnOffDelay/3
  TurnOffDelay/1 -> Logical Operator/1
  Logical Operator/1 -> stBattVltgTmr/1  "CoME_stBattVltgTmr_mp"
  stBattVltg/1 -> EdgeRising/1, Logical Operator/2
  EdgeRising/1 -> TurnOffDelay/1

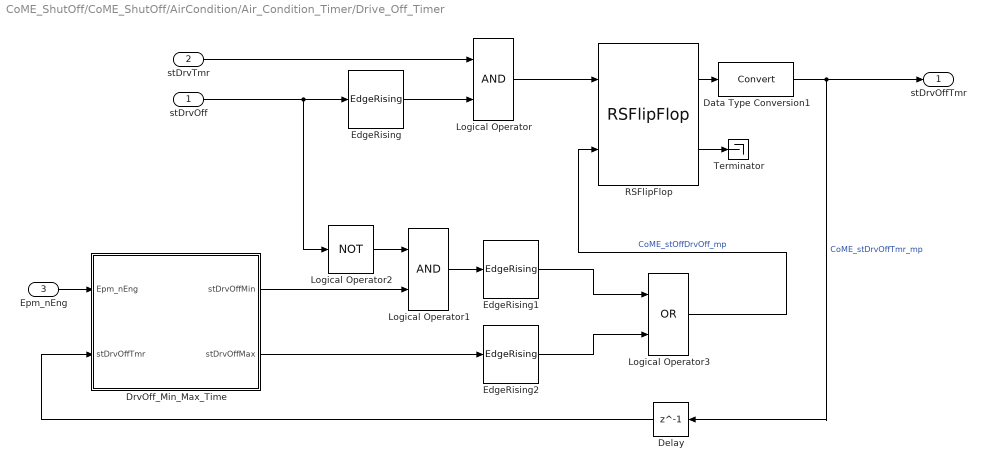
== system CoME_ShutOff/CoME_ShutOff/AirCondition/Air_Condition_Timer/Drive_Off_Timer ==
  stDrvOff : Inport
  stDrvTmr : Inport  Port=2
  Epm_nEng : Inport  Port=3
  Data Type Conversion1 : DataTypeConversion
  Delay : Delay  DelayLength=1  InitialCondition=0
  DrvOff_Min_Max_Time : Subsystem
  EdgeRising : CXLib/EdgeRising
  EdgeRising1 : CXLib/EdgeRising
  EdgeRising2 : CXLib/EdgeRising
  Logical Operator : Logic  OutDataTypeStr=boolean
  Logical Operator1 : Logic  OutDataTypeStr=boolean
  Logical Operator2 : Logic  Operator=NOT  OutDataTypeStr=boolean
  Logical Operator3 : Logic  Operator=OR  OutDataTypeStr=boolean
  RSFlipFlop : CXLib/RSFlipFlop
  Terminator : Terminator
  stDrvOffTmr : Outport
  wires:
  Delay/1 -> DrvOff_Min_Max_Time/2(stDrvOffTmr)
  Data Type Conversion1/1 -> stDrvOffTmr/1, Delay/1  "CoME_stDrvOffTmr_mp"
  Epm_nEng/1 -> DrvOff_Min_Max_Time/1(Epm_nEng)
  Logical Operator3/1 -> RSFlipFlop/2  "CoME_stOffDrvOff_mp"
  EdgeRising1/1 -> Logical Operator3/1
  EdgeRising2/1 -> Logical Operator3/2
  DrvOff_Min_Max_Time/2(stDrvOffMax) -> EdgeRising2/1
  Logical Operator1/1 -> EdgeRising1/1
  Logical Operator2/1 -> Logical Operator1/1
  DrvOff_Min_Max_Time/1(stDrvOffMin) -> Logical Operator1/2
  RSFlipFlop/2 -> Terminator/1
  RSFlipFlop/1 -> Data Type Conversion1/1
  Logical Operator/1 -> RSFlipFlop/1
  stDrvTmr/1 -> Logical Operator/1
  EdgeRising/1 -> Logical Operator/2
  stDrvOff/1 -> EdgeRising/1, Logical Operator2/1

== system CoME_ShutOff/CoME_ShutOff/AirCondition/Air_Condition_Timer/Start_Timer ==
  stStrt : Inport
  Constant1 : Constant  Value=1000  OutDataTypeStr=int16
  Constant2 : Constant  Value=CoME_tiOffStrtAC_C
  Data Store Read : DataStoreRead  DataStoreName=CoME_ShutOff_DT
  Divide : Product  Inputs=**  OutDataTypeStr=Inherit: Inherit via back propagation  SaturateOnIntegerOverflow=on
  TurnOffDelay : CXLib/TurnOffDelay
  stStrtTmr : Outport
  wires:
  Constant1/1 -> Divide/2
  Constant2/1 -> Divide/1
  Divide/1 -> TurnOffDelay/2
  Data Store Read/1 -> TurnOffDelay/3
  stStrt/1 -> TurnOffDelay/1
  TurnOffDelay/1 -> stStrtTmr/1  "CoME_stStrtTmrAC_mp"

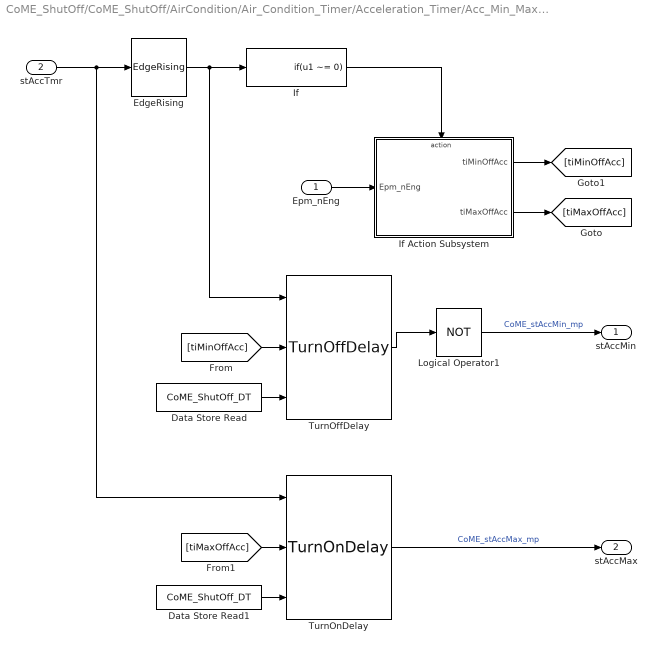
== system CoME_ShutOff/CoME_ShutOff/AirCondition/Air_Condition_Timer/Acceleration_Timer/Acc_Min_Max_Timer ==
  Epm_nEng : Inport
  stAccTmr : Inport  Port=2
  Data Store Read : DataStoreRead  DataStoreName=CoME_ShutOff_DT
  Data Store Read1 : DataStoreRead  DataStoreName=CoME_ShutOff_DT
  EdgeRising : CXLib/EdgeRising
  If : If  IfExpression=u1 ~= 0  ShowElse=off
  If Action Subsystem : Subsystem  TreatAsAtomicUnit=on
  Logical Operator1 : Logic  Operator=NOT  OutDataTypeStr=boolean
  TurnOffDelay : CXLib/TurnOffDelay
  TurnOnDelay : CXLib/TurnOnDelay
  stAccMin : Outport
  stAccMax : Outport  Port=2
  wires:
  Data Store Read1/1 -> TurnOnDelay/3
  Data Store Read/1 -> TurnOffDelay/3
  Logical Operator1/1 -> stAccMin/1  "CoME_stAccMin_mp"
  If Action Subsystem/1(tiMinOffAcc) -> [tiMinOffAcc]
  If Action Subsystem/2(tiMaxOffAcc) -> [tiMaxOffAcc]
  [tiMaxOffAcc] -> TurnOnDelay/2
  [tiMinOffAcc] -> TurnOffDelay/2
  Epm_nEng/1 -> If Action Subsystem/1(Epm_nEng)
  TurnOffDelay/1 -> Logical Operator1/1
  TurnOnDelay/1 -> stAccMax/1  "CoME_stAccMax_mp"
  If/1 -> If Action Subsystem/Action
  EdgeRising/1 -> If/1, TurnOffDelay/1
  stAccTmr/1 -> EdgeRising/1, TurnOnDelay/1

== system CoME_ShutOff/CoME_ShutOff/AirCondition/Air_Condition_Timer/Drive_Off_Timer/DrvOff_Min_Max_Time ==
  Epm_nEng : Inport
  stDrvOffTmr : Inport  Port=2
  Data Store Read : DataStoreRead  DataStoreName=CoME_ShutOff_DT
  Data Store Read1 : DataStoreRead  DataStoreName=CoME_ShutOff_DT
  EdgeRising : CXLib/EdgeRising
  If : If  IfExpression=u1 ~= 0  ShowElse=off
  If Action Subsystem : Subsystem  TreatAsAtomicUnit=on
  Logical Operator1 : Logic  Operator=NOT  OutDataTypeStr=boolean
  TurnOffDelay : CXLib/TurnOffDelay
  TurnOnDelay : CXLib/TurnOnDelay
  stDrvOffMin : Outport
  stDrvOffMax : Outport  Port=2
  wires:
  Data Store Read1/1 -> TurnOnDelay/3
  Data Store Read/1 -> TurnOffDelay/3
  If Action Subsystem/1(tiMinOffDrvOff) -> [tiMinOffDrvOff]
  If Action Subsystem/2(tiMaxOffDrvOff) -> [tiMaxOffDrvOff]
  [tiMaxOffDrvOff] -> TurnOnDelay/2
  [tiMinOffDrvOff] -> TurnOffDelay/2
  Logical Operator1/1 -> stDrvOffMin/1  "CoME_stDrvOffMin_mp"
  TurnOffDelay/1 -> Logical Operator1/1
  TurnOnDelay/1 -> stDrvOffMax/1  "CoME_stDrvOffMax_mp"
  Epm_nEng/1 -> If Action Subsystem/1(Epm_nEng)
  If/1 -> If Action Subsystem/Action
  EdgeRising/1 -> If/1, TurnOffDelay/1
  stDrvOffTmr/1 -> EdgeRising/1, TurnOnDelay/1

== system CoME_ShutOff/CoME_ShutOff/AirCondition/Air_Condition_Timer/Acceleration_Timer/Acc_Min_Max_Timer/If Action Subsystem ==
  Epm_nEng : Inport
  Action Port : ActionPort  ActionType=then
  CoME_tiMaxOffAcc_CUR : Lookup_n-D  NumberOfTableDimensions=1  BreakpointsForDimension1=CoME_tiMaxOffAcc_CURX  BreakpointsForDimension2=HPUn_etaPmp_MAPY  IndexSearchMethod=Linear search  BeginIndexSearchUsingPreviousIndexResult=on  Table=CoME_tiMaxOffAcc_CUR  ExtrapMethod=Clip  UseLastTableValue=on  InternalRulePriority=Speed  OutDataTypeStr=Inherit: Inherit via back propagation  SaturateOnIntegerOverflow=on
  CoME_tiMinOffAcc_CUR : Lookup_n-D  NumberOfTableDimensions=1  BreakpointsForDimension1=CoME_tiMinOffAcc_CURX  BreakpointsForDimension2=HPUn_etaPmp_MAPY  IndexSearchMethod=Linear search  BeginIndexSearchUsingPreviousIndexResult=on  Table=CoME_tiMinOffAcc_CUR  ExtrapMethod=Clip  UseLastTableValue=on  InternalRulePriority=Speed  OutDataTypeStr=Inherit: Inherit via back propagation  SaturateOnIntegerOverflow=on
  tiMinOffAcc : Outport
  tiMaxOffAcc : Outport  Port=2
  wires:
  Epm_nEng/1 -> CoME_tiMinOffAcc_CUR/1, CoME_tiMaxOffAcc_CUR/1
  CoME_tiMaxOffAcc_CUR/1 -> tiMaxOffAcc/1  "CoME_tiMaxOffAcc_mp"
  CoME_tiMinOffAcc_CUR/1 -> tiMinOffAcc/1  "CoME_tiMinOffAcc_mp"

== system CoME_ShutOff/CoME_ShutOff/AirCondition/Air_Condition_Timer/Drive_Off_Timer/DrvOff_Min_Max_Time/If Action Subsystem ==
  Epm_nEng : Inport
  Action Port : ActionPort  ActionType=then
  CoME_tiMaxOffDrvOff_CUR : Lookup_n-D  NumberOfTableDimensions=1  BreakpointsForDimension1=CoME_tiMaxOffDrvOff_CURX  BreakpointsForDimension2=HPUn_etaPmp_MAPY  IndexSearchMethod=Linear search  BeginIndexSearchUsingPreviousIndexResult=on  Table=CoME_tiMaxOffDrvOff_CUR  ExtrapMethod=Clip  UseLastTableValue=on  InternalRulePriority=Speed  OutDataTypeStr=Inherit: Inherit via back propagation  SaturateOnIntegerOverflow=on
  CoME_tiMinOffDrvOff_CUR : Lookup_n-D  NumberOfTableDimensions=1  BreakpointsForDimension1=CoME_tiMinOffDrvOff_CURX  BreakpointsForDimension2=HPUn_etaPmp_MAPY  IndexSearchMethod=Linear search  BeginIndexSearchUsingPreviousIndexResult=on  Table=CoME_tiMinOffDrvOff_CUR  ExtrapMethod=Clip  UseLastTableValue=on  InternalRulePriority=Speed  OutDataTypeStr=Inherit: Inherit via back propagation  SaturateOnIntegerOverflow=on
  tiMinOffDrvOff : Outport
  tiMaxOffDrvOff : Outport  Port=2
  wires:
  CoME_tiMaxOffDrvOff_CUR/1 -> tiMaxOffDrvOff/1  "CoME_tiMaxOffDrvOff_mp"
  CoME_tiMinOffDrvOff_CUR/1 -> tiMinOffDrvOff/1  "CoME_tiMinOffDrvOff_mp"
  Epm_nEng/1 -> CoME_tiMinOffDrvOff_CUR/1, CoME_tiMaxOffDrvOff_CUR/1
